simulink model "voice_tx_system"  (R2025b)
settings: Solver=FixedStepDiscrete  StartTime=0  StopTime=0.5  FixedStep=1/8000  RelTol=1e-3
libraries: dspvision x2, commdigbbndpm3 x2, commfilt2 x2, simulink x2, dspobslib x2, commchan3 x1
settings Model: Creator=zizim  LastModifiedBy=zizim

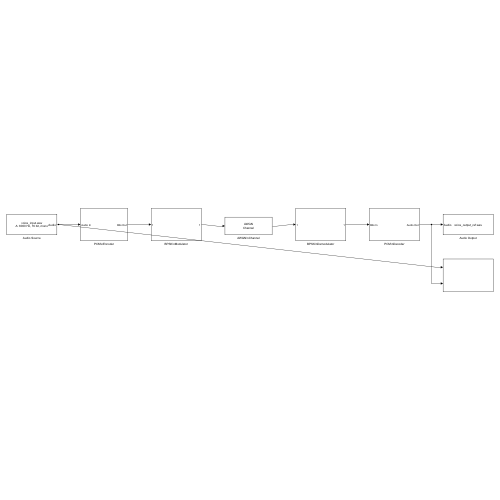
[thumbnail: Simulink's stored preview of the top-level diagram]
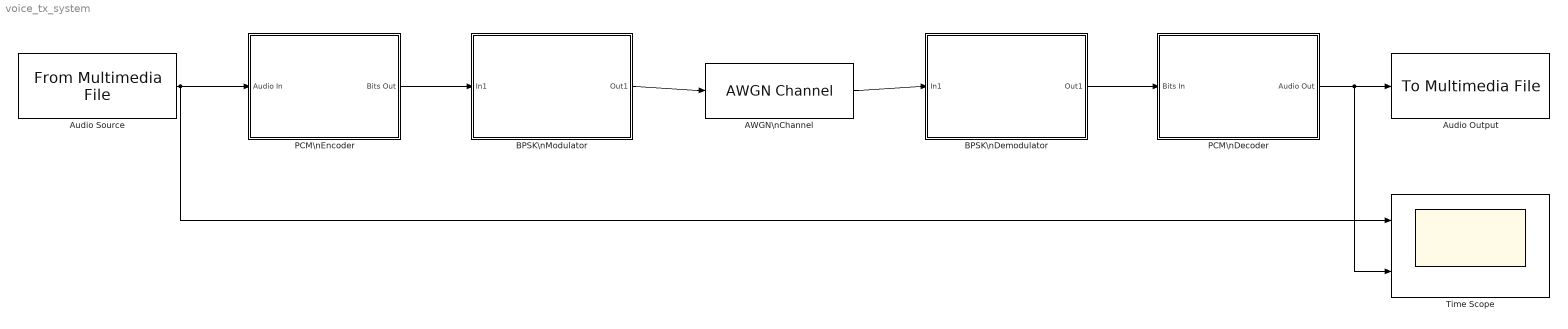
== system voice_tx_system ==
  AWGN\nChannel : commchan3/AWGN Channel  LegacyMode=off  NoiseMethod="Signal to noise ratio  (Eb/No)"  noiseMode="Signal to noise ratio  (Eb/No)"  EbNo=10  EsNo=10  SNR=10  BitsPerSymbol=1  SignalPower=1  SpecifySymbolPeriod=off  SamplesPerSymbol=1  SymbolPeriod=1  VarianceSource=Parameter  Variance=1  RandomStream=Global stream  Seed=67  SimulateUsing=Interpreted execution
  Audio Output : dspvision/To Multimedia File  outputFilename=D:\zizim\Documents\UJN_HW\proj2\voice_output_ref.wav  streamSelection=Audio only  videoCompressor=None (uncompressed)  audioCompressor=None (uncompressed)  imagePorts=One multidimensional signal  fileType=WAV  audioDatatype=16-bit integer  fourcc=RGB  audioBitRate=128  audioQuality=75  videoQuality=75  mj2000CompFactor=10
  Audio Source : dspvision/From Multimedia File  inputFilename=voice_input.wav  readRange=[1 Inf]  loop=on  numPlays=inf  outputStreams=Audio only  videoDataType=single  audioDataType=double  inheritSampleTime=on  userDefinedSampleTime=1/30  noAudioOutput=off  isIntensityVideo=off  fourcc=RGB  colorVideoFormat=One multidimensional signal  outputEOF=off  dataOrg=Column-major  audioFrameSize=80  computeAudioFrameSize=off  outSamplingMode=Sample based
      settings: LibrarySourceBlock=dspsrcs4/From Multimedia File
  BPSK\nDemodulator : Subsystem
  BPSK\nModulator : Subsystem
  PCM\nDecoder : Subsystem
  PCM\nEncoder : Subsystem
  Time Scope : Scope  NumInputPorts=2
      settings: TimeUnits=Metric (based on Time Span)  ActiveDisplayYMinimum=-0.966302738047887  ActiveDisplayYMaximum=1.0150042916762341  YLabel=Amplitude
  wires:
  Audio Source/1 -> PCM\nEncoder/1(Audio In), Time Scope/1
  BPSK\nModulator/1(Out1) -> AWGN\nChannel/1
  AWGN\nChannel/1 -> BPSK\nDemodulator/1(In1)
  BPSK\nDemodulator/1(Out1) -> PCM\nDecoder/1(Bits In)
  PCM\nEncoder/1(Bits Out) -> BPSK\nModulator/1(In1)
  PCM\nDecoder/1(Audio Out) -> Time Scope/2, Audio Output/1

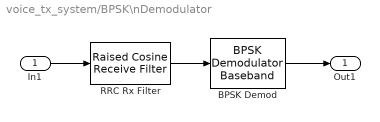
== system voice_tx_system/BPSK\nDemodulator ==
  In1 : Inport
  BPSK Demod : commdigbbndpm3/BPSK Demodulator Baseband  DecType=Hard decision  VarSource=Dialog  Variance=1  Ph=0  outDtype=Inherit via internal rule  derotateFactorWordLen=16  derotateFactorDataTypeStr=Inherit: Same word length as input  derotateFactorLastDataTypeStr=Inherit: Same word length as input
  RRC Rx Filter : commfilt2/Raised Cosine Receive Filter  filtType=Square root  R=0.35  filtSpan=8  N=8  downFactor=8  downOffset=0  filterGain=1  InputProcessing=Columns as channels (frame based)  RateOptions=Enforce single-rate processing  framing=Mute  checkCoeff=off  variableName=rcRxFilt  currentFiltSpan=10  D=5  inputOffset=0  sampMode=Mute  saveAsFlag=0  rateMode=Downsampling  checkGain=Normalized  launchFVT=on  roundingMode=Floor  overflowMode=off  coeffDataTypeStr=Inherit: Same word length as input  coeffMin=[]  coeffMax=[]  coeffLastDataTypeStr=Inherit: Same word length as input  accumDataTypeStr=Inherit: Same as product output  accumLastDataTypeStr=Inherit: Same as product output  outputDataTypeStr=Inherit: Same as accumulator  outputMin=[]  outputMax=[]  outputLastDataTypeStr=Inherit: Same as accumulator
  Out1 : Outport
  wires:
  In1/1 -> RRC Rx Filter/1
  RRC Rx Filter/1 -> BPSK Demod/1
  BPSK Demod/1 -> Out1/1

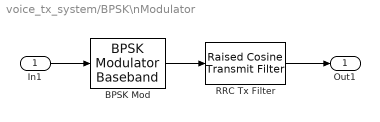
== system voice_tx_system/BPSK\nModulator ==
  In1 : Inport
  BPSK Mod : commdigbbndpm3/BPSK Modulator Baseband  Ph=0  outDtype=double  outWordLen=16  outUDDataType=sfix(16)  outFracLenMode=Best precision  outFracLen=15  outDataTypeStr=double  outLastDataTypeStr=double
  RRC Tx Filter : commfilt2/Raised Cosine Transmit Filter  filtType=Square root  R=0.35  filtSpan=8  N=8  filterGain=1  InputProcessing=Columns as channels (frame based)  RateOptions=Enforce single-rate processing  framing=Mute  checkCoeff=off  variableName=rcTxFilt  checkGain=Normalized  sampMode=Mute  saveAsFlag=0  currentFiltSpan=10  D=(10)/2  launchFVT=on  roundingMode=Floor  overflowMode=off  coeffDataTypeStr=Inherit: Same word length as input  coeffMin=[]  coeffMax=[]  coeffLastDataTypeStr=Inherit: Same word length as input  outputDataTypeStr=Inherit: Same as accumulator  outputMin=[]  outputMax=[]  outputLastDataTypeStr=Inherit: Same as accumulator
  Out1 : Outport
  wires:
  BPSK Mod/1 -> RRC Tx Filter/1
  In1/1 -> BPSK Mod/1
  RRC Tx Filter/1 -> Out1/1

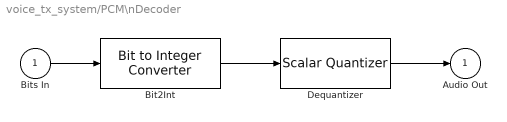
== system voice_tx_system/PCM\nDecoder ==
  Bits In : Inport
  Bit2Int : simulink/Logic and Bit Operations/Bit to Integer Converter  nbits=8  bitOrder=MSB first  signedOutputValues=Unsigned  outDtype=uint8  outDtypeSigned=Inherit via internal rule
      settings: LibrarySourceBlock=|
      | commutil2/Bit to Integer
      | Converter
  Dequantizer : dspobslib/Scalar Quantizer  Qmode=Decoder  QparamSource=Specify via dialog  partitionUnBound=[-0.9921875 -0.984375 -0.9765625 -0.96875 -0.9609375 -0.953125 -0.9453125 -0.9375 -0.9296875 -0.921875 -0.9140625 -0.90625 -0.8984375 -0.890625 -0.8828125 -0.875 -0.8671875 -0.859375 -0.8515625 -0.84375 -0.8359375 -0.828125 -0.8203125 -0.8125 -0.8046875 -0.796875 -0.7890625 -0.78125 -0.7734375 -0.765625 -0.7578125 -0.75 -0.7421875 -0.734375 -0.7265625 -0.71875 -0.7109375 -0.703125 -0.6953125 -0.6875 -0.6796875 -0.671875 -0.6640625 -0.65625 -0.6484375 -0.640625 -0.6328125 -0.625 -0.6171875 -0.609375 -0.6015625 -0.59375 -0.5859375 -0.578125 -0.5703125 -0.5625 -0.5546875 -0.546875 -0.5390625 -0.53125 -0.5234375 -0.515625 -0.5078125 -0.5 -0.4921875 -0.484375 -0.4765625 -0.46875 -0.4609375 -0.453125 -0.4453125 -0.4375 -0.4296875 -0.421875 -0.4140625 -0.40625 -0.3984375 -0.390625 -0.3828125 -0.375 -0.3671875 -0.359375 -0.3515625 -0.34375 -0.3359375 -0.328125 -0.3203125 -0.3125 -0.3046875 -0.296875 -0.2890625 -0.28125 -0.2734375 -0.265625 -0.2578125 -0.25 -0.2421875 -0.234375 -0.2265625 -0.21875 -0.2109375 -0.203125 -0.1953125 -0.1875 -0.1796875 -0.171875 -0.1640625 -0.15625 -0.1484375 -0.140625 -0.1328125 -0.125 -0.1171875 -0.109375 -0.1015625 -0.09375 -0.0859375 -0.078125 -0.0703125 -0.0625 -0.0546875 -0.046875 -0.0390625 -0.03125 -0.0234375 -0.015625 -0.0078125 0 0.0078125 0.015625 0.0234375 0.03125 0.0390625 0.046875 0.0546875 0.0625 0.0703125 0.078125 0.0859375 0.09375 0.1015625 0.109375 0.1171875 0.125 0.1328125 0.140625 0.1484375 0.15625 0.1640625 0.171875 0.1796875 0.1875 0.1953125 0.203125 0.2109375 0.21875 0.2265625 0.234375 0.2421875 0.25 0.2578125 0.265625 0.2734375 0.28125 0.2890625 0.296875 0.3046875 0.3125 0.3203125 0.328125 0.3359375 0.34375 0.3515625 0.359375 0.3671875 0.375 0.3828125 0.390625 0.3984375 0.40625 0.4140625 0.421875 0.4296875 0.4375 0.4453125 0.453125 0.4609375 0.46875 0.4765625 0.484375 0.4921875 0.5 0.5078125 0.515625 0.5234375 0.53125 0.5390625 0.546875 0.5546875 0.5625 0.5703125 0.578125 0.5859375 0.59375 0.6015625 0.609375 0.6171875 0.625 0.6328125 0.640625 0.6484375 0.65625 0.6640625 0.671875 0.6796875 0.6875 0.6953125 0.703125 0.7109375 0.71875 0.7265625 0.734375 0.7421875 0.75 0.7578125 0.765625 0.7734375 0.78125 0.7890625 0.796875 0.8046875 0.8125 0.8203125 0.828125 0.8359375 0.84375 0.8515625 0.859375 0.8671875 0.875 0.8828125 0.890625 0.8984375 0.90625 0.9140625 0.921875 0.9296875 0.9375 0.9453125 0.953125 0.9609375 0.96875 0.9765625 0.984375 0.9921875]  codebook=[-1 -0.9921875 -0.984375 -0.9765625 -0.96875 -0.9609375 -0.953125 -0.9453125 -0.9375 -0.9296875 -0.921875 -0.9140625 -0.90625 -0.8984375 -0.890625 -0.8828125 -0.875 -0.8671875 -0.859375 -0.8515625 -0.84375 -0.8359375 -0.828125 -0.8203125 -0.8125 -0.8046875 -0.796875 -0.7890625 -0.78125 -0.7734375 -0.765625 -0.7578125 -0.75 -0.7421875 -0.734375 -0.7265625 -0.71875 -0.7109375 -0.703125 -0.6953125 -0.6875 -0.6796875 -0.671875 -0.6640625 -0.65625 -0.6484375 -0.640625 -0.6328125 -0.625 -0.6171875 -0.609375 -0.6015625 -0.59375 -0.5859375 -0.578125 -0.5703125 -0.5625 -0.5546875 -0.546875 -0.5390625 -0.53125 -0.5234375 -0.515625 -0.5078125 -0.5 -0.4921875 -0.484375 -0.4765625 -0.46875 -0.4609375 -0.453125 -0.4453125 -0.4375 -0.4296875 -0.421875 -0.4140625 -0.40625 -0.3984375 -0.390625 -0.3828125 -0.375 -0.3671875 -0.359375 -0.3515625 -0.34375 -0.3359375 -0.328125 -0.3203125 -0.3125 -0.3046875 -0.296875 -0.2890625 -0.28125 -0.2734375 -0.265625 -0.2578125 -0.25 -0.2421875 -0.234375 -0.2265625 -0.21875 -0.2109375 -0.203125 -0.1953125 -0.1875 -0.1796875 -0.171875 -0.1640625 -0.15625 -0.1484375 -0.140625 -0.1328125 -0.125 -0.1171875 -0.109375 -0.1015625 -0.09375 -0.0859375 -0.078125 -0.0703125 -0.0625 -0.0546875 -0.046875 -0.0390625 -0.03125 -0.0234375 -0.015625 -0.0078125 0 0.0078125 0.015625 0.0234375 0.03125 0.0390625 0.046875 0.0546875 0.0625 0.0703125 0.078125 0.0859375 0.09375 0.1015625 0.109375 0.1171875 0.125 0.1328125 0.140625 0.1484375 0.15625 0.1640625 0.171875 0.1796875 0.1875 0.1953125 0.203125 0.2109375 0.21875 0.2265625 0.234375 0.2421875 0.25 0.2578125 0.265625 0.2734375 0.28125 0.2890625 0.296875 0.3046875 0.3125 0.3203125 0.328125 0.3359375 0.34375 0.3515625 0.359375 0.3671875 0.375 0.3828125 0.390625 0.3984375 0.40625 0.4140625 0.421875 0.4296875 0.4375 0.4453125 0.453125 0.4609375 0.46875 0.4765625 0.484375 0.4921875 0.5 0.5078125 0.515625 0.5234375 0.53125 0.5390625 0.546875 0.5546875 0.5625 0.5703125 0.578125 0.5859375 0.59375 0.6015625 0.609375 0.6171875 0.625 0.6328125 0.640625 0.6484375 0.65625 0.6640625 0.671875 0.6796875 0.6875 0.6953125 0.703125 0.7109375 0.71875 0.7265625 0.734375 0.7421875 0.75 0.7578125 0.765625 0.7734375 0.78125 0.7890625 0.796875 0.8046875 0.8125 0.8203125 0.828125 0.8359375 0.84375 0.8515625 0.859375 0.8671875 0.875 0.8828125 0.890625 0.8984375 0.90625 0.9140625 0.921875 0.9296875 0.9375 0.9453125 0.953125 0.9609375 0.96875 0.9765625 0.984375 0.9921875]  SearchMethod=Binary  tieBreakRule=Choose the lower index  outQError=off  invalidin=Clip and warn  dtype=off  idtype=int32  cwdtype=double
  Audio Out : Outport
  wires:
  Bits In/1 -> Bit2Int/1
  Bit2Int/1 -> Dequantizer/1
  Dequantizer/1 -> Audio Out/1

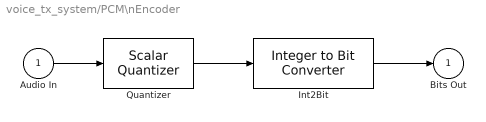
== system voice_tx_system/PCM\nEncoder ==
  Audio In : Inport
  Int2Bit : simulink/Logic and Bit Operations/Integer to Bit Converter  nbits=8  signedInputValues=Unsigned  bitOrder=MSB first  outDtype=uint8
      settings: LibrarySourceBlock=|
      | commutil2/Integer to Bit
      | Converter
  Quantizer : dspobslib/Scalar Quantizer  Qmode=Encoder  QparamSource=Specify via dialog  partitionUnBound=[-0.9921875 -0.984375 -0.9765625 -0.96875 -0.9609375 -0.953125 -0.9453125 -0.9375 -0.9296875 -0.921875 -0.9140625 -0.90625 -0.8984375 -0.890625 -0.8828125 -0.875 -0.8671875 -0.859375 -0.8515625 -0.84375 -0.8359375 -0.828125 -0.8203125 -0.8125 -0.8046875 -0.796875 -0.7890625 -0.78125 -0.7734375 -0.765625 -0.7578125 -0.75 -0.7421875 -0.734375 -0.7265625 -0.71875 -0.7109375 -0.703125 -0.6953125 -0.6875 -0.6796875 -0.671875 -0.6640625 -0.65625 -0.6484375 -0.640625 -0.6328125 -0.625 -0.6171875 -0.609375 -0.6015625 -0.59375 -0.5859375 -0.578125 -0.5703125 -0.5625 -0.5546875 -0.546875 -0.5390625 -0.53125 -0.5234375 -0.515625 -0.5078125 -0.5 -0.4921875 -0.484375 -0.4765625 -0.46875 -0.4609375 -0.453125 -0.4453125 -0.4375 -0.4296875 -0.421875 -0.4140625 -0.40625 -0.3984375 -0.390625 -0.3828125 -0.375 -0.3671875 -0.359375 -0.3515625 -0.34375 -0.3359375 -0.328125 -0.3203125 -0.3125 -0.3046875 -0.296875 -0.2890625 -0.28125 -0.2734375 -0.265625 -0.2578125 -0.25 -0.2421875 -0.234375 -0.2265625 -0.21875 -0.2109375 -0.203125 -0.1953125 -0.1875 -0.1796875 -0.171875 -0.1640625 -0.15625 -0.1484375 -0.140625 -0.1328125 -0.125 -0.1171875 -0.109375 -0.1015625 -0.09375 -0.0859375 -0.078125 -0.0703125 -0.0625 -0.0546875 -0.046875 -0.0390625 -0.03125 -0.0234375 -0.015625 -0.0078125 0 0.0078125 0.015625 0.0234375 0.03125 0.0390625 0.046875 0.0546875 0.0625 0.0703125 0.078125 0.0859375 0.09375 0.1015625 0.109375 0.1171875 0.125 0.1328125 0.140625 0.1484375 0.15625 0.1640625 0.171875 0.1796875 0.1875 0.1953125 0.203125 0.2109375 0.21875 0.2265625 0.234375 0.2421875 0.25 0.2578125 0.265625 0.2734375 0.28125 0.2890625 0.296875 0.3046875 0.3125 0.3203125 0.328125 0.3359375 0.34375 0.3515625 0.359375 0.3671875 0.375 0.3828125 0.390625 0.3984375 0.40625 0.4140625 0.421875 0.4296875 0.4375 0.4453125 0.453125 0.4609375 0.46875 0.4765625 0.484375 0.4921875 0.5 0.5078125 0.515625 0.5234375 0.53125 0.5390625 0.546875 0.5546875 0.5625 0.5703125 0.578125 0.5859375 0.59375 0.6015625 0.609375 0.6171875 0.625 0.6328125 0.640625 0.6484375 0.65625 0.6640625 0.671875 0.6796875 0.6875 0.6953125 0.703125 0.7109375 0.71875 0.7265625 0.734375 0.7421875 0.75 0.7578125 0.765625 0.7734375 0.78125 0.7890625 0.796875 0.8046875 0.8125 0.8203125 0.828125 0.8359375 0.84375 0.8515625 0.859375 0.8671875 0.875 0.8828125 0.890625 0.8984375 0.90625 0.9140625 0.921875 0.9296875 0.9375 0.9453125 0.953125 0.9609375 0.96875 0.9765625 0.984375 0.9921875]  codebook=[-1 -0.9921875 -0.984375 -0.9765625 -0.96875 -0.9609375 -0.953125 -0.9453125 -0.9375 -0.9296875 -0.921875 -0.9140625 -0.90625 -0.8984375 -0.890625 -0.8828125 -0.875 -0.8671875 -0.859375 -0.8515625 -0.84375 -0.8359375 -0.828125 -0.8203125 -0.8125 -0.8046875 -0.796875 -0.7890625 -0.78125 -0.7734375 -0.765625 -0.7578125 -0.75 -0.7421875 -0.734375 -0.7265625 -0.71875 -0.7109375 -0.703125 -0.6953125 -0.6875 -0.6796875 -0.671875 -0.6640625 -0.65625 -0.6484375 -0.640625 -0.6328125 -0.625 -0.6171875 -0.609375 -0.6015625 -0.59375 -0.5859375 -0.578125 -0.5703125 -0.5625 -0.5546875 -0.546875 -0.5390625 -0.53125 -0.5234375 -0.515625 -0.5078125 -0.5 -0.4921875 -0.484375 -0.4765625 -0.46875 -0.4609375 -0.453125 -0.4453125 -0.4375 -0.4296875 -0.421875 -0.4140625 -0.40625 -0.3984375 -0.390625 -0.3828125 -0.375 -0.3671875 -0.359375 -0.3515625 -0.34375 -0.3359375 -0.328125 -0.3203125 -0.3125 -0.3046875 -0.296875 -0.2890625 -0.28125 -0.2734375 -0.265625 -0.2578125 -0.25 -0.2421875 -0.234375 -0.2265625 -0.21875 -0.2109375 -0.203125 -0.1953125 -0.1875 -0.1796875 -0.171875 -0.1640625 -0.15625 -0.1484375 -0.140625 -0.1328125 -0.125 -0.1171875 -0.109375 -0.1015625 -0.09375 -0.0859375 -0.078125 -0.0703125 -0.0625 -0.0546875 -0.046875 -0.0390625 -0.03125 -0.0234375 -0.015625 -0.0078125 0 0.0078125 0.015625 0.0234375 0.03125 0.0390625 0.046875 0.0546875 0.0625 0.0703125 0.078125 0.0859375 0.09375 0.1015625 0.109375 0.1171875 0.125 0.1328125 0.140625 0.1484375 0.15625 0.1640625 0.171875 0.1796875 0.1875 0.1953125 0.203125 0.2109375 0.21875 0.2265625 0.234375 0.2421875 0.25 0.2578125 0.265625 0.2734375 0.28125 0.2890625 0.296875 0.3046875 0.3125 0.3203125 0.328125 0.3359375 0.34375 0.3515625 0.359375 0.3671875 0.375 0.3828125 0.390625 0.3984375 0.40625 0.4140625 0.421875 0.4296875 0.4375 0.4453125 0.453125 0.4609375 0.46875 0.4765625 0.484375 0.4921875 0.5 0.5078125 0.515625 0.5234375 0.53125 0.5390625 0.546875 0.5546875 0.5625 0.5703125 0.578125 0.5859375 0.59375 0.6015625 0.609375 0.6171875 0.625 0.6328125 0.640625 0.6484375 0.65625 0.6640625 0.671875 0.6796875 0.6875 0.6953125 0.703125 0.7109375 0.71875 0.7265625 0.734375 0.7421875 0.75 0.7578125 0.765625 0.7734375 0.78125 0.7890625 0.796875 0.8046875 0.8125 0.8203125 0.828125 0.8359375 0.84375 0.8515625 0.859375 0.8671875 0.875 0.8828125 0.890625 0.8984375 0.90625 0.9140625 0.921875 0.9296875 0.9375 0.9453125 0.953125 0.9609375 0.96875 0.9765625 0.984375 0.9921875]  SearchMethod=Binary  tieBreakRule=Choose the lower index  outQError=off  invalidin=Clip and warn  dtype=off  idtype=int32  cwdtype=double
  Bits Out : Outport
  wires:
  Audio In/1 -> Quantizer/1
  Quantizer/1 -> Int2Bit/1
  Int2Bit/1 -> Bits Out/1
